simulink model "P4_Modelo_4_9_SistRealim"  (R2025b)
settings: Solver=VariableStepAuto  StartTime=0.0  StopTime=10.0  RelTol=1e-3
undefined symbols (not defined in the file): K, k_e, p
settings Model: Creator=Pc24
settings DebuggingCC: UnconnectedInputMsg=warning  UnconnectedOutputMsg=warning  UnconnectedLineMsg=warning
settings ModelReferenceCC: EnableRefExpFcnMdlSchedulingChecks=on
settings RTWCC: GPUComputeCapability=3.5  DLArmComputeVersion=19.05

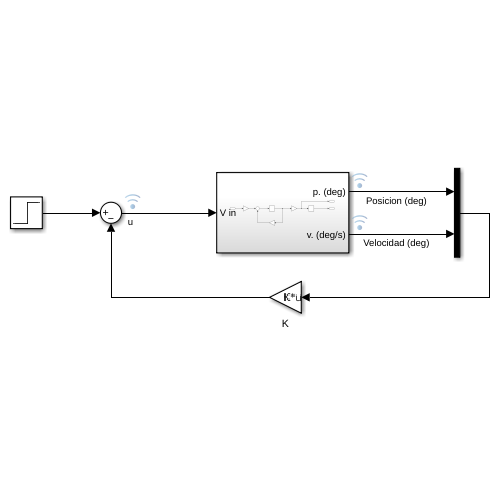
[thumbnail: Simulink's stored preview of the top-level diagram]
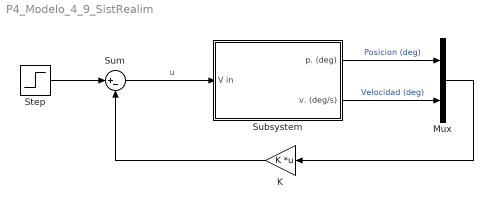
== system P4_Modelo_4_9_SistRealim ==
  K : Gain  Gain=K  Multiplication=Matrix(K*u)
  Mux : Mux  Inputs=2
  Step : Step  SampleTime=0
  Subsystem : Subsystem
  Sum : Sum  Inputs=|+-
  wires:
  Step/1 -> Sum/1
  Sum/1 -> Subsystem/1(V in)  "u"
  Subsystem/1(p. (deg)) -> Mux/1  "Posicion (deg)"
  Subsystem/2(v. (deg/s)) -> Mux/2  "Velocidad (deg)"
  Mux/1 -> K/1
  K/1 -> Sum/2

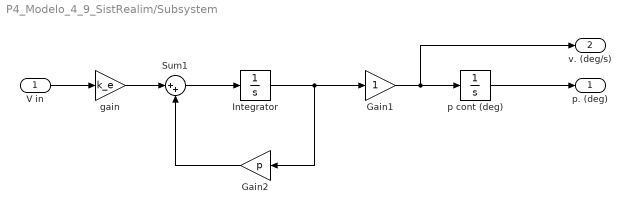
== system P4_Modelo_4_9_SistRealim/Subsystem ==
  V in : Inport
  Gain1 : Gain
  Gain2 : Gain  Gain=p
  Integrator : Integrator
  Sum1 : Sum  Inputs=|++
  gain : Gain  Gain=k_e
  p cont (deg) : Integrator
  p. (deg) : Outport
  v. (deg/s) : Outport  Port=2
  wires:
  V in/1 -> gain/1
  p cont (deg)/1 -> p. (deg)/1
  Integrator/1 -> Gain2/1, Gain1/1
  Gain2/1 -> Sum1/2
  Gain1/1 -> v. (deg/s)/1, p cont (deg)/1
  Sum1/1 -> Integrator/1
  gain/1 -> Sum1/1
